simulink model "simulation"  (R2023a)
settings: Solver=VariableStepAuto  StartTime=0.0  StopTime=0.084  RelTol=1e-3
libraries: spsDistributedParametersLineLib x2, spsThreePhaseSourceLib x2, spsThreePhaseVIMeasurementLib x2, spsThreePhaseFaultLib x1, spspowerguiLib x1
settings Model: SimulationMode=accelerator  Creator=jlhb83  LastModifiedBy=jlhb83
settings SolverCC: DecoupledContinuousIntegration=on  MinimalZcImpactIntegration=on
settings DebuggingCC: ReadBeforeWriteMsg=DisableAll  WriteAfterWriteMsg=DisableAll  WriteAfterReadMsg=DisableAll  MultiTaskDSMMsg=none
settings ModelReferenceCC: UpdateModelReferenceTargets=IfOutOfDate
settings SFSimCC: SFSimEcho=off

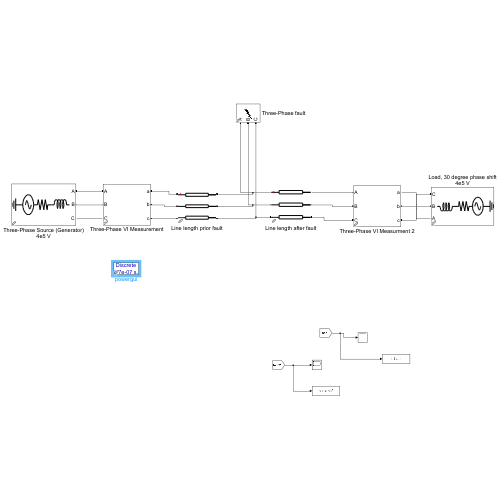
[thumbnail: Simulink's stored preview of the top-level diagram]
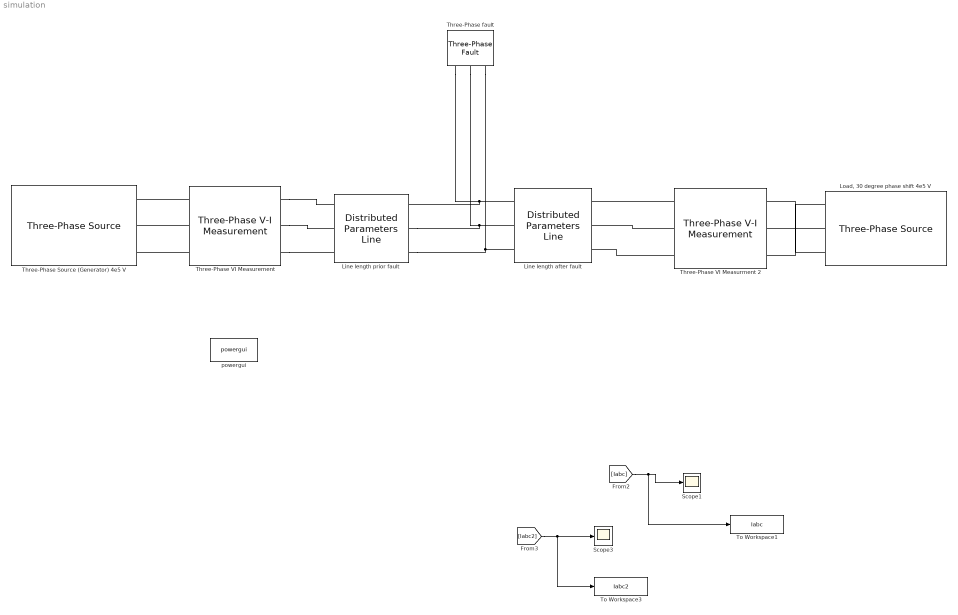
== system simulation ==
  Line length after fault : spsDistributedParametersLineLib/Distributed Parameters Line  Phases=3  Length=15.8404  Frequency=50  Resistance=[0.01273 0.3864]  Inductance=[0.9337e-3 4.1264e-3]  Capacitance=[12.74e-9 7.751e-9]  x1=[-8.978e-05 -4.11600613583729e-10 0 0;-8.911e-05 -4.11570874577877e-10 0 0;-8.844e-05 -4.11541117337519e-10 0 0;-8.777e-05 -4.11511341863975e-10 0 0;-8.71e-05 -4.11481548158562e-10 0 0;-8.643e-05 -4.11451736222603e-10 0 0;-8.576e-05 -4.11421906057416e-10 0 0;-8.509e-05 -4.11392057664324e-10 0 0;-8.442e-05 -4.1136219104465e-10 0 0;-8.375e-05 -4.11332306199716e-10 0 0;-8.308e-05 -4.11302403130846e-10 0 0;-8.241e-05 -4.11272481839366e-10 0 0;-8.174e-05 -4.112425423266e-10 0 0;-8.107e-05 -4.11212584593877e-10 0 0;-8.04e-05 -4.11182608642522e-10 0 0;-7.973e-05 -4.11152614473863e-10 0 0;-7.906e-05 -4.11122602089231e-10 0 0;-7.839e-05 -4.11092571489953e-10 0 0;-7.772e-05 -4.11062522677362e-10 0 0;-7.705e-05 -4.11032455652788e-10 0 0;-7.638e-05 -4.11002370417563e-10 0 0;-7.571e-05 -4.1097226697302e-10 0 0;-7.504e-05 -4.10942145320493e-10 0 0;-7.437e-05 -4.10912005461317e-10 0 0;-7.37e-05 -4.10881847396826e-10 0 0;-7.303e-05 -4.10851671128358e-10 0 0;-7.236e-05 -4.10821476657248e-10 0 0;-7.169e-05 -4.10791263984834e-10 0 0;-7.102e-05 -4.10761033112457e-10 0 0;-7.035e-05 -4.10730784041453e-10 0 0;-6.968e-05 -4.10700516773164e-10 0 0;-6.901e-05 -4.10670231308931e-10 0 0;-6.834e-05 -4.10639927650096e-10 0 0;-6.767e-05 -4.10609605798e-10 0 0;-6.7e-05 -4.10579265753988e-10 0 0;-6.633e-05 -4.10548907519404e-10 0 0;-6.566e-05 -4.10518531095592e-10 0 0;-6.499e-05 -4.10488136483899e-10 0 0;-6.432e-05 -4.10457723685671e-10 0 0;-6.365e-05 -4.10427292702256e-10 0 0;-6.298e-05 -4.10396843535002e-10 0 0;-6.231e-05 -4.10366376185257e-10 0 0;-6.164e-05 -4.10335890654372e-10 0 0;-6.097e-05 -4.10305386943697e-10 0 0;-6.03e-05 -4.10274865054585e-10 0 0;-5.963e-05 -4.10244324988386e-10 0 0;-5.896e-05 -4.10213766746454e-10 0 0;-5.829e-05 -4.10183190330144e-10 0 0;-5.762e-05 -4.10152595740809e-10 0 0;-5.695e-05 -4.10121982979805e-10 0 0;-5.628e-05 -4.10091352048488e-10 0 0;-5.561e-05 -4.10060702948217e-10 0 0;-5.494e-05 -4.10030035680347e-10 114048.640646455 -368046.731840806;-5.427e-05 -4.09999350246239e-10 114126.107064338 -368022.717964994;-5.36e-05 -4.09968646647251e-10 114203.568425904 -367998.687784063;-5.293e-05 -4.09937924884745e-10 114281.02472772 -367974.641299077;-5.226e-05 -4.0990718496008e-10 114358.475966355 -367950.578511103;-5.159e-05 -4.0987642687462e-10 114435.922138377 -367926.499421205;-5.092e-05 -4.09845650629726e-10 114513.363240355 -367902.404030451;-5.025e-05 -4.09814856226762e-10 114590.799268858 -367878.292339908;-4.958e-05 -4.09784043667093e-10 114668.230220456 -367854.164350644;-4.891e-05 -4.09753212952084e-10 114745.656091717 -367830.02006373;-4.824e-05 -4.09722364083101e-10 114823.076879212 -367805.859480233;-4.757e-05 -4.0969149706151e-10 114900.49257951 -367781.682601225;-4.69e-05 -4.09660611888678e-10 114977.903189182 -367757.489427777;-4.623e-05 -4.09629708565976e-10 115055.308704797 -367733.279960961;-4.556e-05 -4.0959878709477e-10 115132.709122926 -367709.054201849;-4.489e-05 -4.09567847476432e-10 115210.104440141 -367684.812151514;-4.422e-05 -4.09536889712333e-10 115287.494653012 -367660.553811031;-4.355e-05 -4.09505913803843e-10 115364.879758111 -367636.279181474;-4.288e-05 -4.09474919752335e-10 115442.259752008 -367611.98826392;-4.221e-05 -4.09443907559183e-10 115519.634631276 -367587.681059443;-4.154e-05 -4.0941287722576e-10 115597.004392486 -367563.357569121;-4.087e-05 -4.09381828753441e-10 115674.369032212 -367539.017794032;-4.02e-05 -4.09350762143602e-10 115751.728547024 -367514.661735254;-3.953e-05 -4.09319677397619e-10 115829.082933496 -367490.289393866;-3.886e-05 -4.0928857451687e-10 115906.432188201 -367465.900770948;-3.819e-05 -4.09257453502732e-10 115983.776307711 -367441.495867581;-3.752e-05 -4.09226314356583e-10 116061.1152886 -367417.074684845;-3.685e-05 -4.09195157079805e-10 116138.449127442 -367392.637223822;-3.618e-05 -4.09163981673777e-10 116215.777820809 -367368.183485596;-3.551e-05 -4.0913278813988e-10 116293.101365277 -367343.71347125;-3.484e-05 -4.09101576479496e-10 116370.41975742 ...(+3451 chars)]  x2=[-8.978e-05 1.02666221623784e-10 0 0;-8.911e-05 1.02551921392494e-10 0 0;-8.844e-05 1.02437616617676e-10 0 0;-8.777e-05 1.02323307304395e-10 0 0;-8.71e-05 1.02208993457716e-10 0 0;-8.643e-05 1.02094675082702e-10 0 0;-8.576e-05 1.01980352184419e-10 0 0;-8.509e-05 1.01866024767932e-10 0 0;-8.442e-05 1.01751692838306e-10 0 0;-8.375e-05 1.01637356400607e-10 0 0;-8.308e-05 1.01523015459899e-10 0 0;-8.241e-05 1.0140867002125e-10 0 0;-8.174e-05 1.01294320089724e-10 0 0;-8.107e-05 1.01179965670389e-10 0 0;-8.04e-05 1.0106560676831e-10 0 0;-7.973e-05 1.00951243388555e-10 0 0;-7.906e-05 1.00836875536189e-10 0 0;-7.839e-05 1.00722503216281e-10 0 0;-7.772e-05 1.00608126433897e-10 0 0;-7.705e-05 1.00493745194105e-10 0 0;-7.638e-05 1.00379359501972e-10 0 0;-7.571e-05 1.00264969362567e-10 0 0;-7.504e-05 1.00150574780956e-10 0 0;-7.437e-05 1.00036175762209e-10 0 0;-7.37e-05 9.99217723113942e-11 0 0;-7.303e-05 9.98073644335796e-11 0 0;-7.236e-05 9.96929521338342e-11 0 0;-7.169e-05 9.95785354172271e-11 0 0;-7.102e-05 9.94641142888275e-11 0 0;-7.035e-05 9.93496887537047e-11 0 0;-6.968e-05 9.92352588169283e-11 0 0;-6.901e-05 9.9120824483568e-11 0 0;-6.834e-05 9.9006385758694e-11 0 0;-6.767e-05 9.88919426473763e-11 0 0;-6.7e-05 9.87774951546852e-11 0 0;-6.633e-05 9.86630432856915e-11 0 0;-6.566e-05 9.85485870454657e-11 0 0;-6.499e-05 9.84341264390789e-11 0 0;-6.432e-05 9.83196614716022e-11 0 0;-6.365e-05 9.82051921481069e-11 0 0;-6.298e-05 9.80907184736645e-11 0 0;-6.231e-05 9.79762404533468e-11 0 0;-6.164e-05 9.78617580922257e-11 0 0;-6.097e-05 9.77472713953732e-11 0 0;-6.03e-05 9.76327803678617e-11 0 0;-5.963e-05 9.75182850147637e-11 0 0;-5.896e-05 9.74037853411517e-11 0 0;-5.829e-05 9.72892813520988e-11 0 0;-5.762e-05 9.71747730526779e-11 0 0;-5.695e-05 9.70602604479623e-11 0 0;-5.628e-05 9.69457435430255e-11 0 0;-5.561e-05 9.6831222342941e-11 0 0;-5.494e-05 9.67166968527827e-11 58454.3229007682 -386814.085997247;-5.427e-05 9.66021670776247e-11 58535.7408287563 -386801.773570522;-5.36e-05 9.6487633022541e-11 58617.1561633386 -386789.444006678;-5.293e-05 9.63730946926062e-11 58698.5689009082 -386777.097306262;-5.226e-05 9.62585520928947e-11 58779.9790378579 -386764.733469821;-5.159e-05 9.61440052284814e-11 58861.386570581 -386752.352497902;-5.092e-05 9.60294541044413e-11 58942.7914954707 -386739.954391053;-5.025e-05 9.59148987258493e-11 59024.1938089204 -386727.539149825;-4.958e-05 9.5800339097781e-11 59105.5935073237 -386715.106774767;-4.891e-05 9.56857752253118e-11 59186.9905870741 -386702.65726643;-4.824e-05 9.55712071135175e-11 59268.3850445653 -386690.190625366;-4.757e-05 9.54566347674738e-11 59349.7768761913 -386677.706852126;-4.69e-05 9.53420581922571e-11 59431.1660783459 -386665.205947265;-4.623e-05 9.52274773929433e-11 59512.5526474233 -386652.687911335;-4.556e-05 9.51128923746092e-11 59593.9365798176 -386640.152744892;-4.489e-05 9.49983031423313e-11 59675.3178719232 -386627.60044849;-4.422e-05 9.48837097011864e-11 59756.6965201345 -386615.031022687;-4.355e-05 9.47691120562516e-11 59838.072520846 -386602.444468038;-4.288e-05 9.46545102126041e-11 59919.4458704524 -386589.840785102;-4.221e-05 9.45399041753213e-11 60000.8165653485 -386577.219974437;-4.154e-05 9.44252939494807e-11 60082.1846019292 -386564.582036601;-4.087e-05 9.43106795401601e-11 60163.5499765895 -386551.926972156;-4.02e-05 9.41960609524375e-11 60244.9126857245 -386539.254781661;-3.953e-05 9.40814381913911e-11 60326.2727257295 -386526.565465679;-3.886e-05 9.3966811262099e-11 60407.6300929999 -386513.85902477;-3.819e-05 9.38521801696399e-11 60488.9847839311 -386501.135459499;-3.752e-05 9.37375449190924e-11 60570.3367949187 -386488.394770429;-3.685e-05 9.36229055155355e-11 60651.6861223586 -386475.636958124;-3.618e-05 9.35082619640481e-11 60733.0327626465 -386462.86202315;-3.551e-05 9.33936142697095e-11 60814.3767121784 -386450.069966072;-3.484e-05 9.32789624375991e-11 60895.7179673504 -386437.260787458;-3.417e-05 9.31643064727966e-11 60977.0565245586 -386424.434487874 ...(+3314 chars)]  x3=[-8.978e-05 3.41534206886925e-11 0 0;-8.911e-05 3.41554821821831e-11 0 0;-8.844e-05 3.41575421624269e-11 0 0;-8.777e-05 3.41596006293326e-11 0 0;-8.71e-05 3.4161657582809e-11 0 0;-8.643e-05 3.4163713022765e-11 0 0;-8.576e-05 3.41657669491095e-11 0 0;-8.509e-05 3.41678193617515e-11 0 0;-8.442e-05 3.41698702606001e-11 0 0;-8.375e-05 3.41719196455644e-11 0 0;-8.308e-05 3.41739675165537e-11 0 0;-8.241e-05 3.41760138734771e-11 0 0;-8.174e-05 3.41780587162441e-11 0 0;-8.107e-05 3.4180102044764e-11 0 0;-8.04e-05 3.41821438589463e-11 0 0;-7.973e-05 3.41841841587006e-11 0 0;-7.906e-05 3.41862229439364e-11 0 0;-7.839e-05 3.41882602145634e-11 0 0;-7.772e-05 3.41902959704914e-11 0 0;-7.705e-05 3.41923302116302e-11 0 0;-7.638e-05 3.41943629378896e-11 0 0;-7.571e-05 3.41963941491796e-11 0 0;-7.504e-05 3.41984238454101e-11 0 0;-7.437e-05 3.42004520264914e-11 0 0;-7.37e-05 3.42024786923334e-11 0 0;-7.303e-05 3.42045038428465e-11 0 0;-7.236e-05 3.42065274779408e-11 0 0;-7.169e-05 3.42085495975268e-11 0 0;-7.102e-05 3.42105702015148e-11 0 0;-7.035e-05 3.42125892898154e-11 0 0;-6.968e-05 3.4214606862339e-11 0 0;-6.901e-05 3.42166229189963e-11 0 0;-6.834e-05 3.4218637459698e-11 0 0;-6.767e-05 3.42206504843548e-11 0 0;-6.7e-05 3.42226619928775e-11 0 0;-6.633e-05 3.4224671985177e-11 0 0;-6.566e-05 3.42266804611642e-11 0 0;-6.499e-05 3.42286874207502e-11 0 0;-6.432e-05 3.42306928638461e-11 0 0;-6.365e-05 3.4232696790363e-11 0 0;-6.298e-05 3.4234699200212e-11 0 0;-6.231e-05 3.42367000933046e-11 0 0;-6.164e-05 3.4238699469552e-11 0 0;-6.097e-05 3.42406973288657e-11 0 0;-6.03e-05 3.42426936711571e-11 0 0;-5.963e-05 3.42446884963379e-11 0 0;-5.896e-05 3.42466818043195e-11 0 0;-5.829e-05 3.42486735950138e-11 0 0;-5.762e-05 3.42506638683324e-11 0 0;-5.695e-05 3.42526526241873e-11 0 0;-5.628e-05 3.42546398624902e-11 0 0;-5.561e-05 3.42566255831531e-11 0 0;-5.494e-05 3.42586097860881e-11 -4138.85297920238 10401.2318366026;-5.427e-05 3.42605924712073e-11 -4141.04220854724 10400.3604326599;-5.36e-05 3.42625736384227e-11 -4143.23125442466 10399.4885679328;-5.293e-05 3.42645532876467e-11 -4145.42011673766 10398.61624246;-5.226e-05 3.42665314187915e-11 -4147.60879538924 10397.7434562802;-5.159e-05 3.42685080317695e-11 -4149.79729028246 10396.8702094319;-5.092e-05 3.42704831264931e-11 -4151.98560132034 10395.9965019538;-5.025e-05 3.42724567028748e-11 -4154.17372840594 10395.1223338847;-4.958e-05 3.42744287608271e-11 -4156.36167144231 10394.2477052634;-4.891e-05 3.42763993002628e-11 -4158.54943033251 10393.3726161284;-4.824e-05 3.42783683210945e-11 -4160.73700497962 10392.4970665187;-4.757e-05 3.42803358232348e-11 -4162.92439528671 10391.621056473;-4.69e-05 3.42823018065968e-11 -4165.11160115688 10390.7445860302;-4.623e-05 3.42842662710933e-11 -4167.29862249322 10389.867655229;-4.556e-05 3.42862292166372e-11 -4169.48545919884 10388.9902641083;-4.489e-05 3.42881906431416e-11 -4171.67211117685 10388.112412707;-4.422e-05 3.42901505505195e-11 -4173.85857833037 10387.2341010639;-4.355e-05 3.42921089386842e-11 -4176.04486056252 10386.3553292181;-4.288e-05 3.42940658075489e-11 -4178.23095777646 10385.4760972083;-4.221e-05 3.42960211570269e-11 -4180.41686987532 10384.5964050737;-4.154e-05 3.42979749870315e-11 -4182.60259676225 10383.7162528531;-4.087e-05 3.42999272974762e-11 -4184.78813834043 10382.8356405855;-4.02e-05 3.43018780882745e-11 -4186.97349451301 10381.95456831;-3.953e-05 3.43038273593399e-11 -4189.15866518318 10381.0730360656;-3.886e-05 3.43057751105862e-11 -4191.34365025413 10380.1910438913;-3.819e-05 3.43077213419269e-11 -4193.52844962905 10379.3085918263;-3.752e-05 3.43096660532759e-11 -4195.71306321114 10378.4256799096;-3.685e-05 3.43116092445471e-11 -4197.89749090361 10377.5423081803;-3.618e-05 3.43135509156543e-11 -4200.08173260969 10376.6584766776;-3.551e-05 3.43154910665114e-11 -4202.2657882326 10375.7741854407;-3.484e-05 3.43174296970326e-11 -4204.44965767558 10374.8894345086;-3.417e-05 3.4319366807132e-11 -4206.63334084187 10374.0042239207;-3.35e-05 ...(+3304 chars)]  x4=[-8.978e-05 -2.65596001617232e-11 0 0;-8.911e-05 -2.65642390062429e-11 0 0;-8.844e-05 -2.65688766738433e-11 0 0;-8.777e-05 -2.65735131643187e-11 0 0;-8.71e-05 -2.65781484774639e-11 0 0;-8.643e-05 -2.65827826130734e-11 0 0;-8.576e-05 -2.65874155709419e-11 0 0;-8.509e-05 -2.65920473508641e-11 0 0;-8.442e-05 -2.65966779526349e-11 0 0;-8.375e-05 -2.66013073760491e-11 0 0;-8.308e-05 -2.66059356209015e-11 0 0;-8.241e-05 -2.66105626869872e-11 0 0;-8.174e-05 -2.66151885741011e-11 0 0;-8.107e-05 -2.66198132820383e-11 0 0;-8.04e-05 -2.66244368105939e-11 0 0;-7.973e-05 -2.6629059159563e-11 0 0;-7.906e-05 -2.66336803287409e-11 0 0;-7.839e-05 -2.66383003179228e-11 0 0;-7.772e-05 -2.6642919126904e-11 0 0;-7.705e-05 -2.66475367554798e-11 0 0;-7.638e-05 -2.66521532034458e-11 0 0;-7.571e-05 -2.66567684705974e-11 0 0;-7.504e-05 -2.666138255673e-11 0 0;-7.437e-05 -2.66659954616394e-11 0 0;-7.37e-05 -2.6670607185121e-11 0 0;-7.303e-05 -2.66752177269706e-11 0 0;-7.236e-05 -2.66798270869839e-11 0 0;-7.169e-05 -2.66844352649567e-11 0 0;-7.102e-05 -2.66890422606848e-11 0 0;-7.035e-05 -2.66936480739642e-11 0 0;-6.968e-05 -2.66982527045907e-11 0 0;-6.901e-05 -2.67028561523603e-11 0 0;-6.834e-05 -2.67074584170692e-11 0 0;-6.767e-05 -2.67120594985134e-11 0 0;-6.7e-05 -2.6716659396489e-11 0 0;-6.633e-05 -2.67212581107922e-11 0 0;-6.566e-05 -2.67258556412193e-11 0 0;-6.499e-05 -2.67304519875667e-11 0 0;-6.432e-05 -2.67350471496307e-11 0 0;-6.365e-05 -2.67396411272076e-11 0 0;-6.298e-05 -2.6744233920094e-11 0 0;-6.231e-05 -2.67488255280863e-11 0 0;-6.164e-05 -2.67534159509812e-11 0 0;-6.097e-05 -2.67580051885752e-11 0 0;-6.03e-05 -2.67625932406651e-11 0 0;-5.963e-05 -2.67671801070476e-11 0 0;-5.896e-05 -2.67717657875194e-11 0 0;-5.829e-05 -2.67763502818774e-11 0 0;-5.762e-05 -2.67809335899184e-11 0 0;-5.695e-05 -2.67855157114395e-11 0 0;-5.628e-05 -2.67900966462375e-11 0 0;-5.561e-05 -2.67946763941096e-11 0 0;-5.494e-05 -2.67992549548528e-11 4751.77923723918 -13193.4950260106;-5.427e-05 -2.68038323282643e-11 4754.55618728798 -13192.4945473836;-5.36e-05 -2.68084085141413e-11 4757.33292668781 -13191.4934842677;-5.293e-05 -2.6812983512281e-11 4760.10945531566 -13190.4918367072;-5.226e-05 -2.68175573224808e-11 4762.8857730485 -13189.4896047465;-5.159e-05 -2.6822129944538e-11 4765.66187976334 -13188.4867884301;-5.092e-05 -2.68267013782499e-11 4768.43777533718 -13187.4833878023;-5.025e-05 -2.68312716234142e-11 4771.21345964703 -13186.4794029076;-4.958e-05 -2.68358406798282e-11 4773.98893256992 -13185.4748337906;-4.891e-05 -2.68404085472897e-11 4776.76419398288 -13184.4696804956;-4.824e-05 -2.68449752255961e-11 4779.53924376296 -13183.4639430673;-4.757e-05 -2.68495407145451e-11 4782.3140817872 -13182.4576215501;-4.69e-05 -2.68541050139346e-11 4785.08870793268 -13181.4507159887;-4.623e-05 -2.68586681235622e-11 4787.86312207645 -13180.4432264277;-4.556e-05 -2.68632300432258e-11 4790.63732409561 -13179.4351529118;-4.489e-05 -2.68677907727233e-11 4793.41131386723 -13178.4264954855;-4.422e-05 -2.68723503118526e-11 4796.18509126843 -13177.4172541936;-4.355e-05 -2.68769086604118e-11 4798.9586561763 -13176.4074290808;-4.288e-05 -2.68814658181988e-11 4801.73200846798 -13175.3970201918;-4.221e-05 -2.68860217850118e-11 4804.50514802057 -13174.3860275714;-4.154e-05 -2.68905765606489e-11 4807.27807471123 -13173.3744512644;-4.087e-05 -2.68951301449083e-11 4810.0507884171 -13172.3622913156;-4.02e-05 -2.68996825375882e-11 4812.82328901533 -13171.3495477698;-3.953e-05 -2.6904233738487e-11 4815.59557638309 -13170.336220672;-3.886e-05 -2.69087837474031e-11 4818.36765039756 -13169.3223100669;-3.819e-05 -2.69133325641348e-11 4821.13951093591 -13168.3078159996;-3.752e-05 -2.69178801884806e-11 4823.91115787535 -13167.292738515;-3.685e-05 -2.69224266202391e-11 4826.68259109307 -13166.277077658;-3.618e-05 -2.69269718592087e-11 4829.45381046629 -13165.2608334737;-3.551e-05 -2.69315159051882e-11 4832.22481587223 -13164.2440060071;-3.484e-05 -2.69360587579762e-11 4834.99560718812 ...(+3449 chars)]  x5=8.95840463783936e-05  V1=[3.176e-08 4.811e+05 4.811e+05;314.2 314.2 314.2;2.009 0.3082 -1.263]  V2=[9.238e-09 4.866e+05 4.866e+05;314.2 314.2 314.2;2.113 0.1934 -1.377]  I1=[1.692e-09 1.742e+04 1.742e+04;314.2 314.2 314.2;-2.491 -2.739 1.973]  I2=[1.679e-09 2.095e+04 2.095e+04;314.2 314.2 314.2;0.6904 0.3759 -1.195]  nHarmo=1  Measurements=None  Decoupling=off  VsMag0=0  VrMag0=0  VsAngle0=0  VrAngle0=0  IsMag0=0  IrMag0=0  IsAngle0=0  IrAngle0=0
      settings: LibrarySourceBlock=sps_lib/Power Grid Elements/Distributed Parameters Line
  Line length prior fault : spsDistributedParametersLineLib/Distributed Parameters Line  Phases=3  Length=4.1596  Frequency=50  Resistance=[0.01273 0.3864]  Inductance=[0.9337e-3 4.1264e-3]  Capacitance=[12.74e-9 7.751e-9]  x1=[-2.412e-05 -1.77319496117804e-10 132153.331624277 -361837.426719071;-2.345e-05 -1.77244729734228e-10 132229.490664917 -361809.602184039;-2.278e-05 -1.77169955497887e-10 132305.643847174 -361781.761619157;-2.211e-05 -1.77095173412091e-10 132381.791167676 -361753.905025659;-2.144e-05 -1.77020383480156e-10 132457.932623048 -361726.03240478;-2.077e-05 -1.76945585705393e-10 132534.068209917 -361698.143757754;-2.01e-05 -1.76870780091118e-10 132610.197924911 -361670.239085817;-1.943e-05 -1.76795966640644e-10 132686.321764655 -361642.318390205;-1.876e-05 -1.76721145357285e-10 132762.439725778 -361614.381672155;-1.809e-05 -1.76646316244358e-10 132838.551804907 -361586.428932905;-1.742e-05 -1.76571479305176e-10 132914.65799867 -361558.460173694;-1.675e-05 -1.76496634543057e-10 132990.758303694 -361530.47539576;-1.608e-05 -1.76421781961315e-10 133066.85271661 -361502.474600343;-1.541e-05 -1.76346921563267e-10 133142.941234044 -361474.457788685;-1.474e-05 -1.76272053352229e-10 133219.023852627 -361446.424962025;-1.407e-05 -1.7619717733152e-10 133295.100568986 -361418.376121607;-1.34e-05 -1.76122293504455e-10 133371.171379753 -361390.311268673;-1.273e-05 -1.76047401874353e-10 133447.236281556 -361362.230404466;-1.206e-05 -1.75972502444532e-10 133523.295271025 -361334.13353023;-1.139e-05 -1.7589759521831e-10 133599.348344791 -361306.020647211;-1.072e-05 -1.75822680199006e-10 133675.395499484 -361277.891756654;-1.005e-05 -1.75747757389938e-10 133751.436731734 -361249.746859804;-9.38e-06 -1.75672826794428e-10 133827.472038174 -361221.58595791;-8.71e-06 -1.75597888415793e-10 133903.501415434 -361193.409052218;-8.04e-06 -1.75522942257355e-10 133979.524860145 -361165.216143977;-7.37e-06 -1.75447988322434e-10 134055.54236894 -361137.007234436;-6.7e-06 -1.7537302661435e-10 134131.553938451 -361108.782324845;-6.03e-06 -1.75298057136425e-10 134207.559565309 -361080.541416454;-5.36e-06 -1.7522307989198e-10 134283.559246148 -361052.284510515;-4.69e-06 -1.75148094884337e-10 134359.552977601 -361024.011608279;-4.02e-06 -1.75073102116818e-10 134435.5407563 -360995.722711;-3.35e-06 -1.74998101592747e-10 134511.522578878 -360967.417819929;-2.68e-06 -1.74923093315445e-10 134587.498441971 -360939.096936323;-2.01e-06 -1.74848077288235e-10 134663.46834221 -360910.760061434;-1.34e-06 -1.74773053514443e-10 134739.432276232 -360882.407196519;-6.7e-07 -1.7469802199739e-10 134815.390240669 -360854.038342834]  x2=[-2.412e-05 -4.08599725842019e-10 117606.810520853 -366925.234034285;-2.345e-05 -4.0856820624359e-10 117684.040799535 -366900.471235859;-2.278e-05 -4.08536668543688e-10 117761.265864267 -366875.692182036;-2.211e-05 -4.0850511274371e-10 117838.485711626 -366850.896873911;-2.144e-05 -4.08473538845055e-10 117915.700338192 -366826.085312585;-2.077e-05 -4.0844194684912e-10 117992.909740544 -366801.257499156;-2.01e-05 -4.08410336757307e-10 118070.113915261 -366776.413434724;-1.943e-05 -4.08378708571014e-10 118147.312858922 -366751.55312039;-1.876e-05 -4.08347062291645e-10 118224.506568108 -366726.676557255;-1.809e-05 -4.083153979206e-10 118301.695039397 -366701.783746422;-1.742e-05 -4.08283715459283e-10 118378.878269371 -366676.874688993;-1.675e-05 -4.08252014909097e-10 118456.05625461 -366651.949386073;-1.608e-05 -4.08220296271446e-10 118533.228991694 -366627.007838764;-1.541e-05 -4.08188559547737e-10 118610.396477204 -366602.050048172;-1.474e-05 -4.08156804739375e-10 118687.558707722 -366577.076015404;-1.407e-05 -4.08125031847767e-10 118764.715679829 -366552.085741565;-1.34e-05 -4.0809324087432e-10 118841.867390106 -366527.079227763;-1.273e-05 -4.08061431820444e-10 118919.013835135 -366502.056475105;-1.206e-05 -4.08029604687547e-10 118996.155011498 -366477.017484701;-1.139e-05 -4.07997759477039e-10 119073.290915778 -366451.962257659;-1.072e-05 -4.07965896190333e-10 119150.421544557 -366426.89079509;-1.005e-05 -4.07934014828838e-10 119227.546894418 -366401.803098104;-9.38e-06 -4.07902115393968e-10 119304.666961943 -366376.699167813;-8.71e-06 -4.07870197887135e-10 119381.781743717 -366351.579005329;-8.04e-06 -4.07838262309755e-10 119458.891236322 -366326.442611765;-7.37e-06 -4.07806308663242e-10 119535.995436342 -366301.289988235;-6.7e-06 -4.07774336949011e-10 119613.094340361 -366276.121135853;-6.03e-06 -4.07742347168479e-10 119690.187944964 -366250.936055734;-5.36e-06 -4.07710339323064e-10 119767.276246734 -366225.734748995;-4.69e-06 -4.07678313414183e-10 119844.359242256 -366200.51721675;-4.02e-06 -4.07646269443256e-10 119921.436928116 -366175.283460119;-3.35e-06 -4.07614207411702e-10 119998.509300898 -366150.033480218;-2.68e-06 -4.07582127320941e-10 120075.576357187 -366124.767278167;-2.01e-06 -4.07550029172395e-10 120152.638093569 -366099.484855084;-1.34e-06 -4.07517912967486e-10 120229.694506631 -366074.186212091;-6.7e-07 -4.07485778707637e-10 120306.745592957 -366048.871350307]  x3=[-2.412e-05 9.49255512679762e-12 -4192.92931433359 10380.4096103141;-2.345e-05 9.48123960267106e-12 -4195.1141596787 10379.526824483;-2.278e-05 9.46992365848145e-12 -4197.29881916074 10378.6435787906;-2.211e-05 9.45860729473016e-12 -4199.4832926829 10377.7598732759;-2.144e-05 9.44729051191855e-12 -4201.66758014841 10376.8757079782;-2.077e-05 9.43597331054799e-12 -4203.85168146049 10375.9910829366;-2.01e-05 9.42465569111991e-12 -4206.03559652238 10375.1059981903;-1.943e-05 9.41333765413571e-12 -4208.21932523732 10374.2204537786;-1.876e-05 9.40201920009685e-12 -4210.40286750855 10373.3344497406;-1.809e-05 9.39070032950478e-12 -4212.58622323934 10372.4479861156;-1.742e-05 9.37938104286098e-12 -4214.76939233296 10371.5610629428;-1.675e-05 9.36806134066695e-12 -4216.95237469268 10370.6736802617;-1.608e-05 9.3567412234242e-12 -4219.13517022178 10369.7858381114;-1.541e-05 9.34542069163427e-12 -4221.31777882356 10368.8975365314;-1.474e-05 9.33409974579871e-12 -4223.50020040131 10368.0087755609;-1.407e-05 9.32277838641909e-12 -4225.68243485835 10367.1195552395;-1.34e-05 9.311456613997e-12 -4227.86448209799 10366.2298756063;-1.273e-05 9.30013442903405e-12 -4230.04634202356 10365.339736701;-1.206e-05 9.28881183203186e-12 -4232.22801453838 10364.4491385628;-1.139e-05 9.27748882349207e-12 -4234.40949954581 10363.5580812313;-1.072e-05 9.26616540391635e-12 -4236.5907969492 10362.666564746;-1.005e-05 9.25484157380638e-12 -4238.77190665189 10361.7745891463;-9.38e-06 9.24351733366386e-12 -4240.95282855726 10360.8821544717;-8.71e-06 9.2321926839905e-12 -4243.13356256869 10359.9892607619;-8.04e-06 9.22086762528803e-12 -4245.31410858954 10359.0959080563;-7.37e-06 9.20954215805822e-12 -4247.49446652323 10358.2020963946;-6.7e-06 9.19821628280283e-12 -4249.67463627314 10357.3078258163;-6.03e-06 9.18689000002365e-12 -4251.85461774269 10356.4130963611;-5.36e-06 9.17556331022248e-12 -4254.03441083529 10355.5179080685;-4.69e-06 9.16423621390116e-12 -4256.21401545437 10354.6222609784;-4.02e-06 9.15290871156153e-12 -4258.39343150336 10353.7261551302;-3.35e-06 9.14158080370543e-12 -4260.5726588857 10352.8295905638;-2.68e-06 9.13025249083477e-12 -4262.75169750485 10351.9325673189;-2.01e-06 9.11892377345143e-12 -4264.93054726425 10351.0350854352;-1.34e-06 9.10759465205732e-12 -4267.10920806738 10350.1371449525;-6.7e-07 9.09626512715439e-12 -4269.28767981772 10349.2387459105]  x4=[-2.412e-05 2.07054393275433e-11 5109.30850485992 -13074.0445668331;-2.345e-05 2.07107307547212e-11 5112.06030425491 -13072.9688356943;-2.278e-05 2.07160212643173e-11 5114.81187716183 -13071.8925253621;-2.211e-05 2.07213108560973e-11 5117.56322345878 -13070.8156358842;-2.144e-05 2.07265995298267e-11 5120.31434302387 -13069.7381673084;-2.077e-05 2.07318872852714e-11 5123.0652357352 -13068.6601196823;-2.01e-05 2.07371741221969e-11 5125.81590147089 -13067.5814930538;-1.943e-05 2.07424600403691e-11 5128.56634010909 -13066.5022874706;-1.876e-05 2.07477450395538e-11 5131.31655152793 -13065.4225029805;-1.809e-05 2.07530291195168e-11 5134.06653560557 -13064.3421396314;-1.742e-05 2.07583122800241e-11 5136.81629222016 -13063.2611974711;-1.675e-05 2.07635945208415e-11 5139.56582124988 -13062.1796765476;-1.608e-05 2.07688758417351e-11 5142.31512257292 -13061.0975769087;-1.541e-05 2.07741562424707e-11 5145.06419606747 -13060.0148986024;-1.474e-05 2.07794357228146e-11 5147.81304161173 -13058.9316416767;-1.407e-05 2.07847142825328e-11 5150.56165908391 -13057.8478061795;-1.34e-05 2.07899919213914e-11 5153.31004836224 -13056.7633921589;-1.273e-05 2.07952686391566e-11 5156.05820932496 -13055.678399663;-1.206e-05 2.08005444355946e-11 5158.80614185029 -13054.5928287397;-1.139e-05 2.08058193104717e-11 5161.55384581651 -13053.5066794371;-1.072e-05 2.08110932635542e-11 5164.30132110187 -13052.4199518035;-1.005e-05 2.08163662946083e-11 5167.04856758465 -13051.332645887;-9.38e-06 2.08216384034006e-11 5169.79558514312 -13050.2447617356;-8.71e-06 2.08269095896974e-11 5172.54237365559 -13049.1562993977;-8.04e-06 2.08321798532652e-11 5175.28893300037 -13048.0672589214;-7.37e-06 2.08374491938704e-11 5178.03526305575 -13046.977640355;-6.7e-06 2.08427176112797e-11 5180.78136370008 -13045.8874437468;-6.03e-06 2.08479851052596e-11 5183.52723481168 -13044.7966691451;-5.36e-06 2.08532516755767e-11 5186.2728762689 -13043.7053165981;-4.69e-06 2.08585173219977e-11 5189.01828795009 -13042.6133861543;-4.02e-06 2.08637820442893e-11 5191.76346973363 -13041.5208778621;-3.35e-06 2.08690458422183e-11 5194.50842149788 -13040.4277917697;-2.68e-06 2.08743087155514e-11 5197.25314312123 -13039.3341279258;-2.01e-06 2.08795706640555e-11 5199.99763448208 -13038.2398863786;-1.34e-06 2.08848316874974e-11 5202.74189545884 -13037.1450671767;-6.7e-07 2.08900917856441e-11 5205.48592592991 -13036.0496703687]  x5=2.35242670207549e-05  V1=[3.068e-08 4.81e+05 4.81e+05;314.2 314.2 314.2;2.039 0.32 -1.251]  V2=[3.176e-08 4.811e+05 4.811e+05;314.2 314.2 314.2;2.026 0.3188 -1.252]  I1=[7.871e-09 1.742e+04 1.742e+04;314.2 314.2 314.2;0.1369 -2.728 1.984]  I2=[5.905e-09 2.096e+04 2.096e+04;314.2 314.2 314.2;-2.617 0.3972 -1.174]  nHarmo=1  Measurements=None  Decoupling=off  VsMag0=0  VrMag0=0  VsAngle0=0  VrAngle0=0  IsMag0=0  IrMag0=0  IsAngle0=0  IrAngle0=0
      settings: LibrarySourceBlock=sps_lib/Power Grid Elements/Distributed Parameters Line
  "Load, 30 degree phase shift 4e5 V" : spsThreePhaseSourceLib/Three-Phase Source  InternalConnection=Yg  VoltagePhases=off  Voltage=400e3  PhaseAngle=-30  Voltage_phases=[25e3 25e3 25e3]/sqrt(3)  PhaseAngles_phases=[0 -120 +120]  Frequency=50  NonIdealSource=on  SpecifyImpedance=off  Resistance=0.8929  Inductance=16.58e-3  ShortCircuitLevel=100e6  BaseVoltage=400e3  XRratio=7  BusType=swing  Pref=10e3  Qref=0  Prefabc=[10e3, 10e3, 10e3]  Qrefabc=[0, 0, 0]  Qmin=-inf  Qmax=inf
  Scope1 : Scope
  Scope3 : Scope
  Three-Phase Source (Generator) 4e5 V : spsThreePhaseSourceLib/Three-Phase Source  InternalConnection=Yg  VoltagePhases=off  Voltage=400e3  PhaseAngle=0  Voltage_phases=[25e3 25e3 25e3]/sqrt(3)  PhaseAngles_phases=[0 -120 +120]  Frequency=50  NonIdealSource=on  SpecifyImpedance=off  Resistance=0.8929  Inductance=16.58e-3  ShortCircuitLevel=100e6  BaseVoltage=400e3  XRratio=7  BusType=swing  Pref=10e3  Qref=0  Prefabc=[10e3, 10e3, 10e3]  Qrefabc=[0, 0, 0]  Qmin=-inf  Qmax=inf
  Three-Phase VI Measurement : spsThreePhaseVIMeasurementLib/Three-Phase V-I Measurement  VoltageMeasurement=no  SetLabelV=off  LabelV=Vabc  Vpu=off  VpuLL=off  CurrentMeasurement=yes  SetLabelI=on  LabelI=Iabc  Ipu=on  Pbase=831.4e6  Vbase=400e3  OutputType=Complex  PhasorSimulation=off  PSBequivalent=0
  Three-Phase VI Measurment 2 : spsThreePhaseVIMeasurementLib/Three-Phase V-I Measurement  VoltageMeasurement=no  SetLabelV=on  LabelV=Vabc2  Vpu=on  VpuLL=off  CurrentMeasurement=yes  SetLabelI=on  LabelI=Iabc2  Ipu=on  Pbase=831.4e6  Vbase=400e3  OutputType=Complex  PhasorSimulation=off  PSBequivalent=0
  Three-Phase fault : spsThreePhaseFaultLib/Three-Phase Fault  InitialStates=0  FaultA=on  FaultB=on  FaultC=on  GroundFault=on  SwitchTimes=[0.028]  External=off  SwitchStatus=NaN  FaultResistance=5  GroundResistance=0.01  SnubberResistance=1e6  SnubberCapacitance=inf  Measurements=None
  To Workspace1 : ToWorkspace  VariableName=Iabc  SaveFormat=Timeseries  SampleTime=-1
  To Workspace3 : ToWorkspace  VariableName=Iabc2  SaveFormat=Timeseries  SampleTime=-1
  powergui : spspowerguiLib/powergui  Priority=1  SimulationMode=Discrete  SampleTime=6.7e-7  frequency=20e3  Iterations=50  frequencyindice=0  Pbase=100e6  ErrMax=1e-4  UnitsV=kV  UnitsW=MW  buscounter=0  FunctionMessages=off  echomessages=off  EnableUseOfTLC=off  CurrentSourceSwitches=off  DisableSnubberDevices=off  DisableRonSwitches=off  DisableVfSwitches=off  DisplayEquations=off  AutomaticDiscreteSolvers=off  SolverType=Tustin/Backward Euler (TBE)  Interpol=off  ExternalGateDelay=off  methode=off  Ts=100  x0status=blocks  SPID=on  SwTol=0  HookPort=off  NonlinearTolerance=1e-4  nMaxIteration=100  ContinueOnMaxIteration=off  RestoreLinks=warning  ResistiveCurrentMeasurement=off  Frange=[0:2:500]  Ylog=off  Xlog=on  ShowGrid=off  save=off  variable=ZData  structure=0  ZoomFFT=off  StartTime=0.0  cycles=1  DisplayStyle=1  fundamental=60  FreqAxis=off  MaxFrequency=1000  frequencyindicesteady=1  RmsSteady=1  display=off
  wires:
  [Iabc2] -> To Workspace3/1, Scope3/1
  [Iabc] -> To Workspace1/1, Scope1/1
  connections:
  Line length after fault/LConn1 -- Three-Phase fault/LConn1 -- Line length prior fault/RConn1
  Line length prior fault/RConn2 -- Three-Phase fault/LConn2 -- Line length after fault/LConn2
  Line length prior fault/RConn3 -- Three-Phase fault/LConn3 -- Line length after fault/LConn3
  Three-Phase VI Measurment 2/LConn3 -- Line length after fault/RConn3
  Three-Phase VI Measurment 2/LConn2 -- Line length after fault/RConn2
  Three-Phase VI Measurment 2/LConn1 -- Line length after fault/RConn1
  "Load, 30 degree phase shift 4e5 V"/RConn2 -- Three-Phase VI Measurment 2/RConn2
  "Load, 30 degree phase shift 4e5 V"/RConn1 -- Three-Phase VI Measurment 2/RConn1
  "Load, 30 degree phase shift 4e5 V"/RConn3 -- Three-Phase VI Measurment 2/RConn3
  Three-Phase VI Measurement/RConn2 -- Line length prior fault/LConn2
  Three-Phase VI Measurement/RConn1 -- Line length prior fault/LConn1
  Three-Phase VI Measurement/RConn3 -- Line length prior fault/LConn3
  Three-Phase VI Measurement/LConn1 -- Three-Phase Source (Generator) 4e5 V/RConn1
  Three-Phase VI Measurement/LConn2 -- Three-Phase Source (Generator) 4e5 V/RConn2
  Three-Phase VI Measurement/LConn3 -- Three-Phase Source (Generator) 4e5 V/RConn3
